simulink model "mpc_controller"  (R2023b)
settings: Solver=VariableStepAuto  StartTime=0.0  StopTime=10.0  RelTol=1e-3
values from neighbouring files (symbols this model uses):
  TP = TP9    [dissipativity_analysis.m]
settings Model: Creator=fabioschneider  LastModifiedBy=fabioschneider

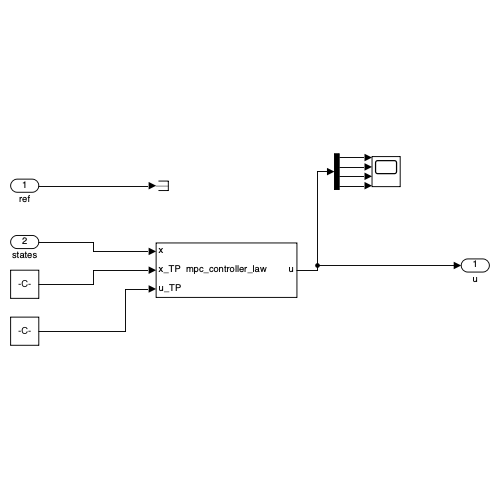
[thumbnail: Simulink's stored preview of the top-level diagram]
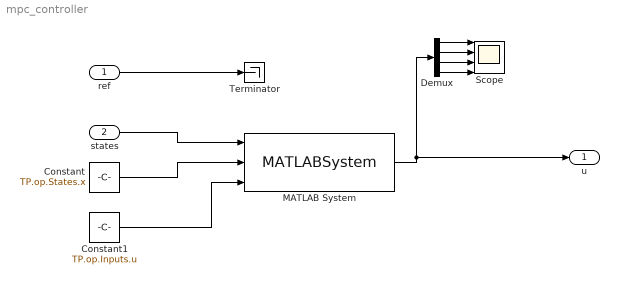
== system mpc_controller ==
  ref : Inport  PortDimensions=[4;1]
  states : Inport  Port=2  PortDimensions=[9,1]
  Constant : Constant  Value=TP.op.States.x
  Constant1 : Constant  Value=TP.op.Inputs.u
  Demux : Demux
  MATLAB System : MATLABSystem  System=mpc_controller_law  SimulateUsing=Interpreted execution
      mask Type: mpc_controller_law
      mask Display:
      | disp('mpc_controller_law');
      | port_label('input',1,'x');
      | port_label('input',2,'x_TP');
      | port_label('input',3,'u_TP');
      | port_label('output',1,'u');
  Scope : Scope  NumInputPorts=4
  Terminator : Terminator
  u : Outport
  wires:
  Demux/2 -> Scope/2
  Demux/4 -> Scope/4
  states/1 -> MATLAB System/1
  ref/1 -> Terminator/1
  Demux/3 -> Scope/3
  Constant/1 -> MATLAB System/2
  Demux/1 -> Scope/1
  MATLAB System/1 -> Demux/1, u/1
  Constant1/1 -> MATLAB System/3
